simulink model "SeesawModelYeni"  (R2017b)
settings: Solver=ode3  StartTime=0.0  StopTime=10  FixedStep=0.01  RelTol=1e-3  EnableMultiTasking=on
values from neighbouring files (symbols this model uses):
  b = 1    [SeesawModel_parameters.m]
  g = 9.8    [SeesawModel_parameters.m]
  J = 1    [SeesawModel_parameters.m]
  K = 1    [SeesawModel_parameters.m]
  L = 1    [SeesawModel_parameters.m]
  md = 1    [SeesawModel_parameters.m]
  mp = 1    [SeesawModel_parameters.m]
  mr = 1    [SeesawModel_parameters.m]
  R = 1    [SeesawModel_parameters.m]
  rwheel = 1    [SeesawModel_parameters.m]
  testStep = 1    [SeesawModel_parameters.m]
  x1initial = 1    [SeesawModel_parameters.m]
  x2 = 1    [SeesawModel_parameters.m]
settings Model: Creator=Administrator  LastModifiedBy=Orhun
settings DataIOCC: LimitDataPoints=on  SaveFormat=Array
settings OptimizationCC: LifeSpan=inf
settings DebuggingCC: SFUnexpectedBacktrackingDiag=warning  SFNoUnconditionalDefaultTransitionDiag=warning  SFExecutionAtInitializationDiag=none
settings HardwareCC: ProdBitPerPointer=32  ProdBitPerSizeT=32  ProdBitPerPtrDiffT=32  ProdLargestAtomicFloat=None  ProdIntDivRoundTo=Undefined  ProdEndianess=Unspecified  ProdWordSize=32  ProdHWDeviceType=32-bit Generic
settings ModelReferenceCC: PropagateSignalLabelsOutOfModel=off
settings CodeAppCC: StateflowObjectComments=on
settings GRTTargetCC: TargetLangStandard=C89/C90 (ANSI)  GeneratePreprocessorConditionals=Disable all
settings ConfigComp: CovMetricSettings=dw  CovHtmlReporting=on  CovSaveCumulativeToWorkspaceVar=on  CovSaveSingleToWorkspaceVar=on  CovExternalEMLEnable=off

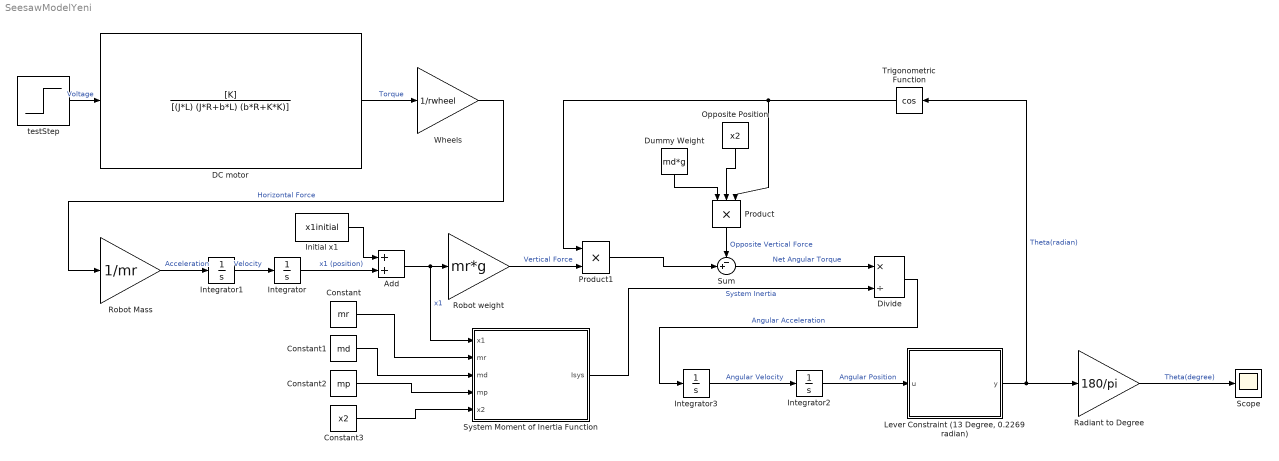
== system SeesawModelYeni ==
  Add : Sum
  Constant : Constant  Value=mr
  Constant1 : Constant  Value=md
  Constant2 : Constant  Value=mp
  Constant3 : Constant  Value=x2
  DC motor : TransferFcn  Numerator=[K]  Denominator=[(J*L) (J*R+b*L) (b*R+K*K)]
  Divide : Product  Inputs=*/
  Dummy Weight : Constant  Value=md*g
  Initial x1 : Constant  Value=x1initial
  Integrator : Integrator
  Integrator1 : Integrator
  Integrator2 : Integrator
  Integrator3 : Integrator  UpperSaturationLimit=100
  "Lever Constraint (13 Degree, 0.2269 radian)" : MATLAB Function  TreatAsAtomicUnit=on
  Opposite Position : Constant  Value=x2
  Product : Product  Inputs=3
  Product1 : Product
  Radiant to Degree : Gain  Gain=180/pi
  Robot Mass : Gain  Gain=1/mr
  Robot weight : Gain  Gain=mr*g
  Scope : Scope
  Sum : Sum  Inputs=-+|
  System Moment of Inertia Function : MATLAB Function  TreatAsAtomicUnit=on
  Trigonometric Function : Trigonometry  Operator=cos
  Wheels : Gain  Gain=1/rwheel
  testStep : Step  After=testStep  SampleTime=0
  wires:
  testStep/1 -> DC motor/1  "Voltage"
  DC motor/1 -> Wheels/1  "Torque"
  Wheels/1 -> Robot Mass/1  "Horizontal Force"
  Robot Mass/1 -> Integrator1/1  "Acceleration"
  Integrator1/1 -> Integrator/1  "Velocity"
  Dummy Weight/1 -> Product/1
  Opposite Position/1 -> Product/2
  Product/1 -> Sum/1  "Opposite Vertical Force"
  Robot weight/1 -> Product1/2  "Vertical Force"
  Sum/1 -> Divide/1  "Net Angular Torque"
  Divide/1 -> Integrator3/1  "Angular Acceleration"
  Integrator3/1 -> Integrator2/1  "Angular Velocity"
  Integrator2/1 -> "Lever Constraint (13 Degree, 0.2269 radian)"/1(u)  "Angular Position"
  System Moment of Inertia Function/1(Isys) -> Divide/2  "System Inertia"
  Constant/1 -> System Moment of Inertia Function/2(mr)
  Constant3/1 -> System Moment of Inertia Function/5(x2)
  Constant2/1 -> System Moment of Inertia Function/4(mp)
  Constant1/1 -> System Moment of Inertia Function/3(md)
  "Lever Constraint (13 Degree, 0.2269 radian)"/1(y) -> Radiant to Degree/1, Trigonometric Function/1  "Theta(radian)"
  Radiant to Degree/1 -> Scope/1  "Theta(degree)"
  Product1/1 -> Sum/2
  Integrator/1 -> Add/2  "x1 (position)"
  Add/1 -> System Moment of Inertia Function/1(x1), Robot weight/1  "x1"
  Initial x1/1 -> Add/1
  Trigonometric Function/1 -> Product1/1, Product/3

== matlab function SeesawModelYeni/Lever Constraint (13 Degree, 0.2269 radian) ==
  data: u input; y output
function y = leverConstraint(u)
if u>=0.2269    %0.2269=13*(pi/180)
    y=0.2269;
elseif u<=-0.2269
    y=-0.2269;
else
    y=u;
end

== matlab function SeesawModelYeni/System Moment of Inertia Function ==
  data: x1 input; Isys output; mr input; md input; mp input; x2 input
function Isys = Inertia(x1, mr, md, mp, x2)
M=mr+md+mp;
Mmasses=mr+md;
Isys=M*((Mmasses*((mr*x1+md*x2)/Mmasses))/M)^2;
